simulink model "pend_MPC"  (R2018b)
settings: Solver=FixedStepAuto  StartTime=0.0  StopTime=30  FixedStep=h  RelTol=1e-3  EnableMultiTasking=on
PreLoadFcn:
  | hwinit
StartFcn:
  | hwinit
values from neighbouring files (symbols this model uses):
  adingain = [1, 1]    [hwinit.m]
  adinoffs = [-0.2676;-0.1653]    [hwinit.m]
  d_cart = X(1)    [main.m]
  d_pend = X_2(1)    [main.m]    (also in pend_par.m = x(1))
  daoutgain = [0.9]    [hwinit.m]
  daoutoffs = [0]    [hwinit.m]
  h = 0.01    [calib.m]    (also in main.m = 0.001; pend_par.m)
  Km = X(2)    [main.m]
  mc = X(3)    [main.m]
  mp = X_2(2)    [main.m]    (also in pend_par.m = x(2))
  option = 1    [main.m]
  T_final = 40    [main.m]
  x_init = [Pos_Pendulum.data(1),0,Angle_Pendulum.data(1),0]    [main.m]
undefined symbols (not defined in the file or in its folder): Advantech, angle_bound, angle_real, DiscIntNeverNeededParam, Discrete, dsys, K, kalman, l, PCI, pend, Time
libraries: simulink x2, sldrtlib x2, ctrlSharedLib x1, mpclib x1
settings Model: Creator=zhidayat  LastModifiedBy=dvanhanswijk
settings DataIOCC: LimitDataPoints=on  SaveFormat=Array
settings OptimizationCC: ExpressionDepthLimit=2147483647  LifeSpan=inf
settings DebuggingCC: AllowSymbolicDim=off  StateNameClashWarn=warning  StrictBusMsg=ErrorOnBusTreatedAsVector  SFUnexpectedBacktrackingDiag=warning  SFNoUnconditionalDefaultTransitionDiag=warning  SFExecutionAtInitializationDiag=none
settings HardwareCC: ProdBitPerPointer=32  ProdBitPerSizeT=32  ProdBitPerPtrDiffT=32  ProdLargestAtomicFloat=None  ProdIntDivRoundTo=Undefined  ProdEndianess=Unspecified  ProdWordSize=32  ProdHWDeviceType=32-bit Generic
settings ModelReferenceCC: PropagateSignalLabelsOutOfModel=off
settings SFSimCC: SimUseLocalCustomCode=off
settings RTWCC: RTWUseLocalCustomCode=off
settings CodeAppCC: StateflowObjectComments=on
settings GRTTargetCC: TargetLangStandard=C89/C90 (ANSI)  GeneratePreprocessorConditionals=Disable all  CombineOutputUpdateFcns=off  GRTInterface=on
settings ConfigComp: CovMetricSettings=dw  CovHtmlReporting=on  CovSaveCumulativeToWorkspaceVar=on  CovSaveSingleToWorkspaceVar=on  CovExternalEMLEnable=off

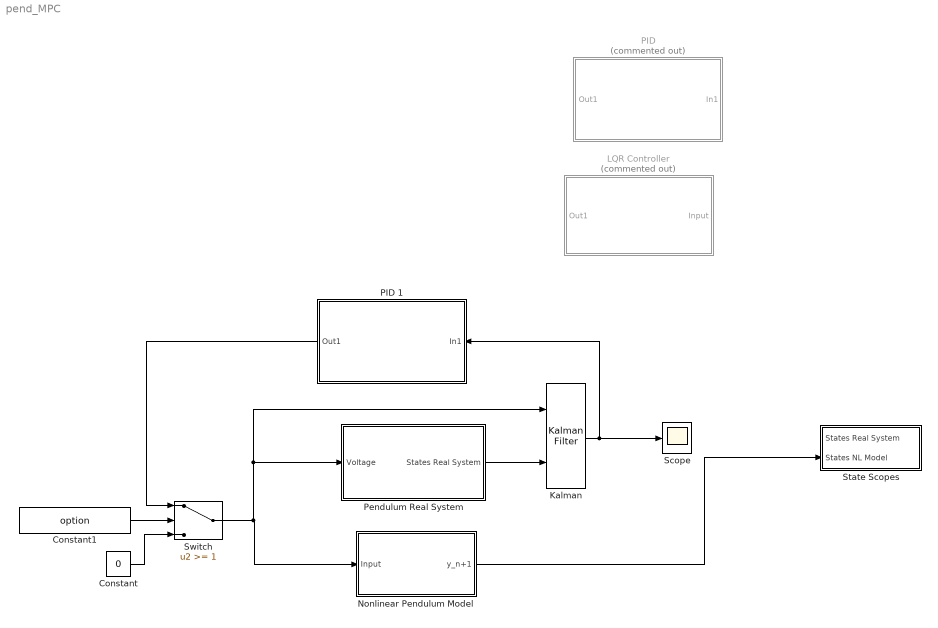
== system pend_MPC ==
  Constant : Constant  Value=0
  Constant1 : Constant  Value=option
  "Kalman " : ctrlSharedLib/Kalman Filter  TimeDomain=Discrete-Time  UseCurrentEstimator=on  ModelSource=Individual A, B, C, D matrices  ModelSourceVariable=ss(0.95,1,1,0,1)  A=dsys.A  B=dsys.B  C=dsys.C  D=dsys.D  NumberOfStates=4  NumberOfInputs=1  NumberOfOutputs=2  InitialEstimateSource=Dialog  X0=x_init  P0=10  UseK=off  UseGH=off  NumberOfProcessNoiseInputs=1  G=1  TimeInvariantG=on  H=0  TimeInvariantH=on  Q=kalman.Q  TimeInvariantQ=on  R=kalman.R  TimeInvariantR=on  N=0  TimeInvariantN=on  AddInputPort=on  AddEnablePort=off  OutputEstimatedY=off  OutputP=off  Ts=h
      settings: SourceProductBaseCode=CT
  LQR Controller : Subsystem  Commented=on
  Nonlinear Pendulum Model : Subsystem
  "PID " : Subsystem  Commented=on
  PID 1 : Subsystem
  "Pendulum Real System " : Subsystem
  Scope : Scope
  "State Scopes " : Subsystem
  Switch : Switch  Threshold=1
  wires:
  Nonlinear Pendulum Model/1(y_n+1) -> "State Scopes "/2(States NL Model)
  Constant/1 -> Switch/3
  Constant1/1 -> Switch/2
  "Pendulum Real System "/1(States Real System) -> "Kalman "/2
  PID 1/1(Out1) -> Switch/1
  Switch/1 -> Nonlinear Pendulum Model/1(Input), "Pendulum Real System "/1(Voltage), "Kalman "/1
  "Kalman "/1 -> Scope/1, PID 1/1(In1)

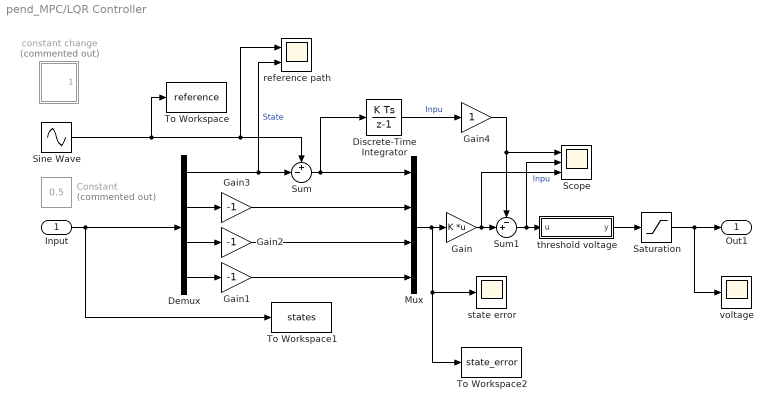
== system pend_MPC/LQR Controller ==
  Input : Inport
  Constant : Constant  Commented=on  Value=0.5
  Demux : Demux
  Discrete-Time Integrator : DiscreteIntegrator  gainval=1  SampleTime=h  ICPrevOutput=DiscIntNeverNeededParam  ICPrevScaledInput=DiscIntNeverNeededParam
  Gain : Gain  Gain=K  Multiplication=Matrix(K*u)
  Gain1 : Gain  Gain=-1
  Gain2 : Gain  Gain=-1
  Gain3 : Gain  Gain=-1
  Gain4 : Gain
  Mux : Mux
  Saturation : Saturate  UpperLimit=1  LowerLimit=-1
  Scope : Scope  NumInputPorts=3
  Sine Wave : Sin  Amplitude=0.1  Bias=0.5  SampleTime=h
  Sum : Sum  Inputs=+-|
  Sum1 : Sum  Inputs=-+|
  To Workspace : ToWorkspace  VariableName=reference  SaveFormat=Timeseries  SampleTime=-1
  To Workspace1 : ToWorkspace  VariableName=states  SaveFormat=Timeseries  SampleTime=-1
  To Workspace2 : ToWorkspace  VariableName=state_error  SaveFormat=Timeseries  SampleTime=-1
  "constant change " : Subsystem  Commented=on
  reference path : Scope  NumInputPorts=2
  state error : Scope
  threshold voltage : MATLAB Function  TreatAsAtomicUnit=on
  voltage : Scope
  Out1 : Outport
  wires:
  Input/1 -> To Workspace1/1, Demux/1
  Demux/2 -> Gain3/1
  Mux/1 -> Gain/1, To Workspace2/1, state error/1
  Demux/1 -> reference path/2, Sum/2  "State"
  Demux/3 -> Gain2/1
  Demux/4 -> Gain1/1
  threshold voltage/1(y) -> Saturation/1
  Sine Wave/1 -> To Workspace/1, reference path/1, Sum/1
  Gain/1 -> Scope/3, Sum1/2  "Inpu"
  Sum1/1 -> Scope/2, threshold voltage/1(u)
  Saturation/1 -> voltage/1, Out1/1
  Sum/1 -> Discrete-Time Integrator/1, Mux/1
  Gain3/1 -> Mux/2
  Gain2/1 -> Mux/3
  Gain1/1 -> Mux/4
  Discrete-Time Integrator/1 -> Gain4/1  "Inpu"
  Gain4/1 -> Scope/1, Sum1/1

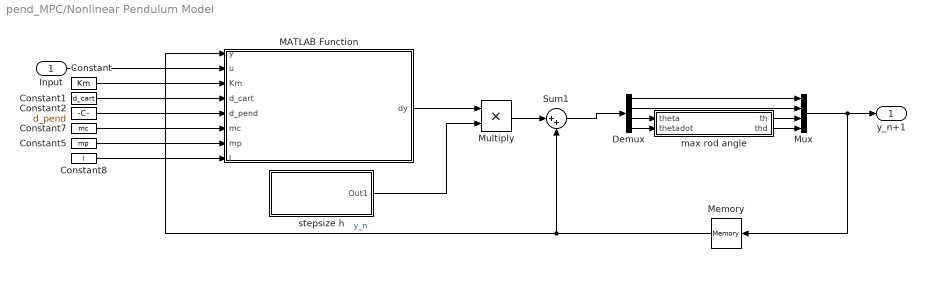
== system pend_MPC/Nonlinear Pendulum Model ==
  Input : Inport
  Constant : Constant  Value=Km
  Constant1 : Constant  Value=d_cart
  Constant2 : Constant  Value=d_pend
  Constant5 : Constant  Value=mp
  Constant7 : Constant  Value=mc
  Constant8 : Constant  Value=l  SampleTime=h
  Demux : Demux
  MATLAB Function : MATLAB Function  TreatAsAtomicUnit=on
  Memory : Memory  InitialCondition=x_init
  Multiply : Product
  Mux : Mux
  Sum1 : Sum  Inputs=|++
  max rod angle : MATLAB Function  TreatAsAtomicUnit=on
  stepsize h : Subsystem
  y_n+1 : Outport
  wires:
  Multiply/1 -> Sum1/1
  Memory/1 -> MATLAB Function/1(y), Sum1/2  "y_n"
  stepsize h/1(Out1) -> Multiply/2
  Constant/1 -> MATLAB Function/3(Km)
  Constant1/1 -> MATLAB Function/4(d_cart)
  Demux/2 -> Mux/2
  Demux/1 -> Mux/1
  Input/1 -> MATLAB Function/2(u)
  Constant2/1 -> MATLAB Function/5(d_pend)
  MATLAB Function/1(dy) -> Multiply/1
  Constant5/1 -> MATLAB Function/7(mp)
  Constant7/1 -> MATLAB Function/6(mc)
  Constant8/1 -> MATLAB Function/8(l)
  Demux/3 -> max rod angle/1(theta)
  Demux/4 -> max rod angle/2(thetadot)
  max rod angle/1(th) -> Mux/3
  max rod angle/2(thd) -> Mux/4
  Sum1/1 -> Demux/1
  Mux/1 -> Memory/1, y_n+1/1

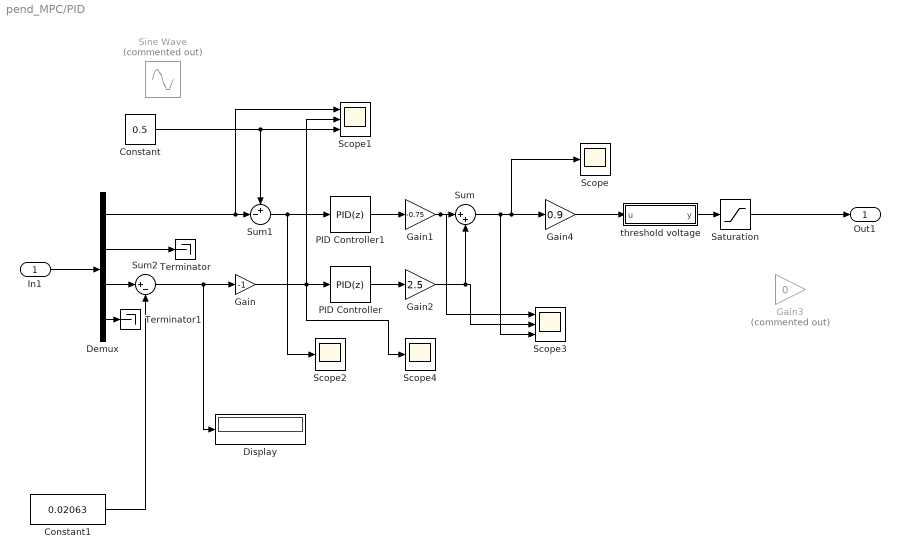
== system pend_MPC/PID  ==
  In1 : Inport
  Constant : Constant  Value=0.5
  Constant1 : Constant  Value=0.02063
  Demux : Demux
  Display : Display
  Gain : Gain  Gain=-1
  Gain1 : Gain  Gain=-0.75
  Gain2 : Gain  Gain=2.5
  Gain3 : Gain  Commented=on  Gain=0
  Gain4 : Gain  Gain=0.9
  PID Controller : simulink/Continuous/PID Controller  Controller=PID  Form=Parallel  TimeDomain=Discrete-time  SampleTime=h  IntegratorMethod=Forward Euler  FilterMethod=Forward Euler  ControllerParametersSource=internal  P=30  I=0  D=0.015  UseFilter=on  N=100  TunerSelectOption=Transfer Function Based (PID Tuner App)  InitialConditionSource=internal  InitialConditionForIntegrator=0  InitialConditionForFilter=0  DifferentiatorICPrevScaledInput=0  ExternalReset=none  TrackingMode=off  Kt=1  LimitOutput=off  UpperSaturationLimit=inf  LowerSaturationLimit=-inf  LinearizeAsGain=on  AntiWindupMode=none  Kb=1  POutMin=[]  POutMax=[]  IOutMin=[]  IOutMax=[]  DOutMin=[]  DOutMax=[]  NOutMin=[]  NOutMax=[]  SumOutMin=[]  SumOutMax=[]  SaturationOutMin=[]  SaturationOutMax=[]  PParamMin=[]  PParamMax=[]  IParamMin=[]  IParamMax=[]  DParamMin=[]  DParamMax=[]  NParamMin=[]  NParamMax=[]  KbParamMin=[]  KbParamMax=[]  KtParamMin=[]  KtParamMax=[]  KbOutMin=[]  KbOutMax=[]  KtOutMin=[]  KtOutMax=[]  IntegratorOutMin=[]  IntegratorOutMax=[]  FilterOutMin=[]  FilterOutMax=[]  SumI1OutMin=[]  SumI1OutMax=[]  SumI2OutMin=[]  SumI2OutMax=[]  SumI3OutMin=[]  SumI3OutMax=[]  SumI4OutMin=[]  SumI4OutMax=[]  SumDOutMin=[]  SumDOutMax=[]  DifferentiatorOutMin=[]  DifferentiatorOutMax=[]  FilterDiffOutCoefMin=[]  FilterDiffOutCoefMax=[]  ReciprocalOutMin=[]  ReciprocalOutMax=[]  SumDenOutMin=[]  SumDenOutMax=[]  SumNumOutMin=[]  SumNumOutMax=[]  DivideOutMin=[]  DivideOutMax=[]  IntegratorContinuousStateAttributes=''  IntegratorStateMustResolveToSignalObject=off  IntegratorRTWStateStorageClass=Auto  FilterContinuousStateAttributes=''  FilterStateMustResolveToSignalObject=off  FilterRTWStateStorageClass=Auto  ParallelPVariant=InternalParameters  IdealPVariant=Disabled  IVariant=InternalParameters  DVariant=InternalParameters  IntegratorVariant=Discrete  SatVariant=Disabled  AWVariant=Passthrough  PCopyVariant=Disabled  TRVariant=Disabled  FdbkBlocksVariant=Forward  IdealPFdbkVariant=Disabled  SatFdbkVariant=Disabled  DerivativeFilterVariant=ForwardEulerFilter  NVariant=InternalParameters  NCopyVariant=Disabled  FilterICVariant=InternalICsFilter  IntegratorICVariant=InternalICs  ExternalResetVariant=Disabled  TRSumVariant=Passthrough  SumFdbkVariant=Disabled  SumVariant=Sum_PID
  PID Controller1 : simulink/Continuous/PID Controller  Controller=PID  Form=Parallel  TimeDomain=Discrete-time  SampleTime=h  IntegratorMethod=Forward Euler  FilterMethod=Forward Euler  ControllerParametersSource=internal  P=13  I=0.75  D=0.75  UseFilter=on  N=100  TunerSelectOption=Transfer Function Based (PID Tuner App)  InitialConditionSource=internal  InitialConditionForIntegrator=0  InitialConditionForFilter=0  DifferentiatorICPrevScaledInput=0  ExternalReset=none  TrackingMode=off  Kt=1  LimitOutput=off  UpperSaturationLimit=inf  LowerSaturationLimit=-inf  LinearizeAsGain=on  AntiWindupMode=none  Kb=1  POutMin=[]  POutMax=[]  IOutMin=[]  IOutMax=[]  DOutMin=[]  DOutMax=[]  NOutMin=[]  NOutMax=[]  SumOutMin=[]  SumOutMax=[]  SaturationOutMin=[]  SaturationOutMax=[]  PParamMin=[]  PParamMax=[]  IParamMin=[]  IParamMax=[]  DParamMin=[]  DParamMax=[]  NParamMin=[]  NParamMax=[]  KbParamMin=[]  KbParamMax=[]  KtParamMin=[]  KtParamMax=[]  KbOutMin=[]  KbOutMax=[]  KtOutMin=[]  KtOutMax=[]  IntegratorOutMin=[]  IntegratorOutMax=[]  FilterOutMin=[]  FilterOutMax=[]  SumI1OutMin=[]  SumI1OutMax=[]  SumI2OutMin=[]  SumI2OutMax=[]  SumI3OutMin=[]  SumI3OutMax=[]  SumI4OutMin=[]  SumI4OutMax=[]  SumDOutMin=[]  SumDOutMax=[]  DifferentiatorOutMin=[]  DifferentiatorOutMax=[]  FilterDiffOutCoefMin=[]  FilterDiffOutCoefMax=[]  ReciprocalOutMin=[]  ReciprocalOutMax=[]  SumDenOutMin=[]  SumDenOutMax=[]  SumNumOutMin=[]  SumNumOutMax=[]  DivideOutMin=[]  DivideOutMax=[]  IntegratorContinuousStateAttributes=''  IntegratorStateMustResolveToSignalObject=off  IntegratorRTWStateStorageClass=Auto  FilterContinuousStateAttributes=''  FilterStateMustResolveToSignalObject=off  FilterRTWStateStorageClass=Auto  ParallelPVariant=InternalParameters  IdealPVariant=Disabled  IVariant=InternalParameters  DVariant=InternalParameters  IntegratorVariant=Discrete  SatVariant=Disabled  AWVariant=Passthrough  PCopyVariant=Disabled  TRVariant=Disabled  FdbkBlocksVariant=Forward  IdealPFdbkVariant=Disabled  SatFdbkVariant=Disabled  DerivativeFilterVariant=ForwardEulerFilter  NVariant=InternalParameters  NCopyVariant=Disabled  FilterICVariant=InternalICsFilter  IntegratorICVariant=InternalICs  ExternalResetVariant=Disabled  TRSumVariant=Passthrough  SumFdbkVariant=Disabled  SumVariant=Sum_PID
  Saturation : Saturate  UpperLimit=1  LowerLimit=-1
  Scope : Scope
  Scope1 : Scope  NumInputPorts=3
  Scope2 : Scope
  Scope3 : Scope  NumInputPorts=3
  Scope4 : Scope
  Sine Wave : Sin  Commented=on  Amplitude=0.15  Bias=0.5  Frequency=0.5  SampleTime=h
  Sum : Sum  Inputs=|++
  Sum1 : Sum  Inputs=+-|
  Sum2 : Sum  Inputs=|+-
  Terminator : Terminator
  Terminator1 : Terminator
  threshold voltage : MATLAB Function  TreatAsAtomicUnit=on
  Out1 : Outport
  wires:
  Demux/2 -> Terminator/1
  Demux/4 -> Terminator1/1
  PID Controller1/1 -> Gain1/1
  Sum/1 -> Scope3/3, Scope/1, Gain4/1
  In1/1 -> Demux/1
  PID Controller/1 -> Gain2/1
  Demux/1 -> Scope1/1, Sum1/2
  Constant/1 -> Scope1/3, Sum1/1
  Sum1/1 -> Scope2/1, PID Controller1/1
  Gain1/1 -> Scope3/1, Sum/1
  Gain2/1 -> Scope3/2, Sum/2
  threshold voltage/1(y) -> Saturation/1
  Sum2/1 -> Gain/1, Display/1
  Saturation/1 -> Out1/1
  Demux/3 -> Sum2/1
  Constant1/1 -> Sum2/2
  Gain/1 -> Scope1/2, PID Controller/1, Scope4/1
  Gain4/1 -> threshold voltage/1(u)

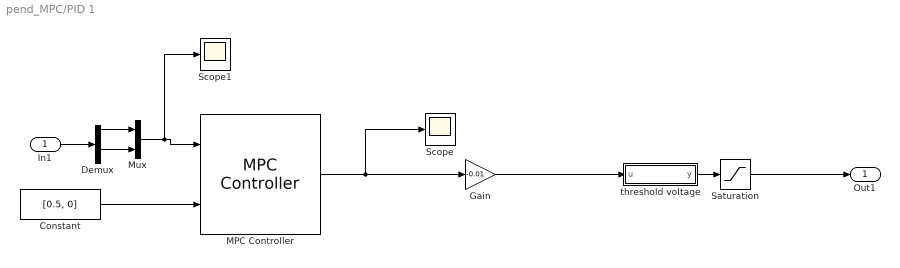
== system pend_MPC/PID 1 ==
  In1 : Inport
  Constant : Constant  Value=[0.5, 0]
  Demux : Demux
  Gain : Gain  Gain=-0.01
  MPC Controller : mpclib/MPC Controller  SCDEnableBlockLinearizationSpecification=on  mpcobj=MPCOBJ  is_multiple=0  enable_value=0  return_u0=off  updateMPCinCallerWorkspace=on  md_inport=off  mv_inport=off  return_cost=off  return_mvseq=off  return_qpstatus=off  return_xseq=off  return_state=off  return_ovseq=off  state_inport=off  umin_inport=off  umax_inport=off  ymin_inport=off  ymax_inport=off  cc_inport=off  ywt_inport=off  uwt_inport=off  duwt_inport=off  rhoeps_inport=off  uref_inport=off  n_ts=0.001  n_p=10  n_mv=1  n_md=0  n_ud=0  n_mo=2  n_uo=0  BlockDataType=double  SampleTimeInherited=off  switch_inport=off
  Mux : Mux  Inputs=2
  Saturation : Saturate  UpperLimit=1  LowerLimit=-1
  Scope : Scope
  Scope1 : Scope
  threshold voltage : MATLAB Function  TreatAsAtomicUnit=on
  Out1 : Outport
  wires:
  threshold voltage/1(y) -> Saturation/1
  Saturation/1 -> Out1/1
  Constant/1 -> MPC Controller/2
  Gain/1 -> threshold voltage/1(u)
  In1/1 -> Demux/1
  Demux/1 -> Mux/1
  Demux/3 -> Mux/2
  Mux/1 -> Scope1/1, MPC Controller/1
  MPC Controller/1 -> Scope/1, Gain/1

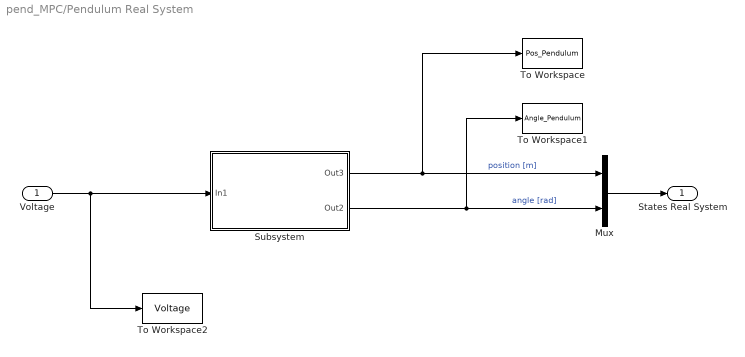
== system pend_MPC/Pendulum Real System  ==
  Voltage : Inport
  Mux : Mux  Inputs=2
  Subsystem : Subsystem  InitFcn=hwinit  StartFcn=hwinit  mask{h=h}
      mask prompts: h "Sample time"
      mask init:
      | hwinit
      mask Display: disp('Pendulum');
  To Workspace : ToWorkspace  VariableName=Pos_Pendulum  SaveFormat=Timeseries  SampleTime=-1
  To Workspace1 : ToWorkspace  VariableName=Angle_Pendulum  SaveFormat=Timeseries  SampleTime=-1
  To Workspace2 : ToWorkspace  VariableName=Voltage  SaveFormat=Timeseries  SampleTime=-1
  States Real System : Outport
  wires:
  Voltage/1 -> To Workspace2/1, Subsystem/1(In1)
  Subsystem/1(Out3) -> To Workspace/1, Mux/1  "position [m]"
  Subsystem/2(Out2) -> Mux/2, To Workspace1/1  "angle [rad]"
  Mux/1 -> States Real System/1

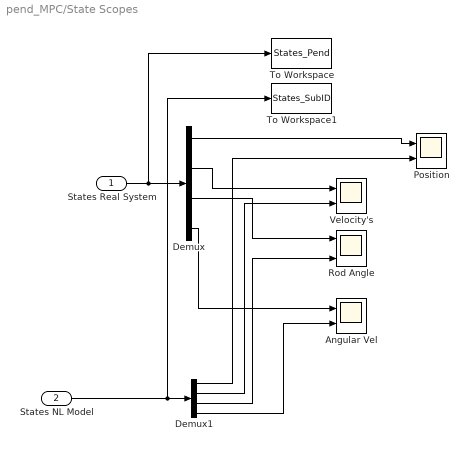
== system pend_MPC/State Scopes  ==
  States Real System : Inport
  States NL Model : Inport  Port=2
  "Angular Vel " : Scope  NumInputPorts=2
  Demux : Demux
  Demux1 : Demux
  Position : Scope  NumInputPorts=2
  Rod Angle : Scope  NumInputPorts=2
  To Workspace : ToWorkspace  VariableName=States_Pend  SaveFormat=Timeseries  SampleTime=-1
  To Workspace1 : ToWorkspace  VariableName=States_SubID  SaveFormat=Timeseries  SampleTime=h
  Velocity's : Scope  NumInputPorts=2
  wires:
  States Real System/1 -> To Workspace/1, Demux/1
  Demux/1 -> Position/1
  States NL Model/1 -> To Workspace1/1, Demux1/1
  Demux1/2 -> Velocity's/2
  Demux/2 -> Velocity's/1
  Demux/3 -> Rod Angle/1
  Demux1/3 -> Rod Angle/2
  Demux/4 -> "Angular Vel "/1
  Demux1/4 -> "Angular Vel "/2
  Demux1/1 -> Position/2

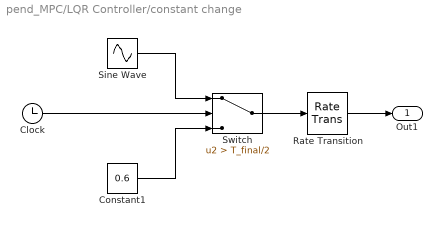
== system pend_MPC/LQR Controller/constant change  ==
  Clock : Clock
  Constant1 : Constant  Value=0.6
  Rate Transition : RateTransition  OutPortSampleTime=h
  Sine Wave : Sin  Amplitude=0.2  Bias=0.5  SampleTime=h
  Switch : Switch  Criteria=u2 > Threshold  Threshold=T_final/2
  Out1 : Outport
  wires:
  Sine Wave/1 -> Switch/1
  Constant1/1 -> Switch/3
  Clock/1 -> Switch/2
  Switch/1 -> Rate Transition/1
  Rate Transition/1 -> Out1/1

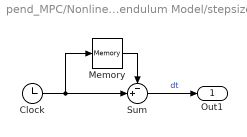
== system pend_MPC/Nonlinear Pendulum Model/stepsize h ==
  Clock : Clock
  Memory : Memory
  Sum : Sum  Inputs=-+|
  Out1 : Outport
  wires:
  Memory/1 -> Sum/1
  Sum/1 -> Out1/1  "dt"
  Clock/1 -> Memory/1, Sum/2

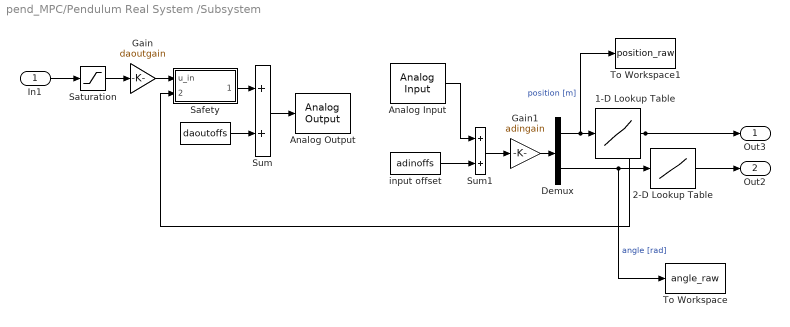
== system pend_MPC/Pendulum Real System /Subsystem ==
  In1 : Inport
  " " : Constant  Value=daoutoffs
  1-D Lookup Table : Lookup_n-D  NumberOfTableDimensions=1  BreakpointsForDimension1=pend  Table=real  InternalRulePriority=Speed  RndMeth=Simplest  InputSameDT=on
  2-D Lookup Table : Lookup_n-D  NumberOfTableDimensions=1  BreakpointsForDimension1=angle_real  BreakpointsForDimension2=[1:3]  Table=angle_bound  InternalRulePriority=Speed  RndMeth=Simplest  InputSameDT=on
  Analog Input : sldrtlib/Analog Input  SampleTime=h  MaxMissedTicks=ticklost  ShowMissedTicks=off  YieldWhenWaiting=on  DrvName=Advantech/PCI-1711  DrvAddress=4294967295  DrvOptions=zeros(1,0)  Channels=adinchannels  RangeMode=2  VoltRange=1  DataType=1
      settings: AttributesFormatString=Advantech\nPCI-1711 [auto]  SourceProductName=Simulink Desktop Real-Time
  Analog Output : sldrtlib/Analog Output  SampleTime=h  MaxMissedTicks=ticklost  ShowMissedTicks=off  YieldWhenWaiting=off  DrvName=Advantech/PCI-1711  DrvAddress=4294967295  DrvOptions=zeros(1,0)  Channels=daoutchannels  RangeMode=2  VoltRange=2  InitialValue=0  FinalValue=0
      settings: AttributesFormatString=Advantech\nPCI-1711 [auto]  SourceProductName=Simulink Desktop Real-Time
  Demux : Demux  Outputs=2
  Gain : Gain  Gain=daoutgain  SaturateOnIntegerOverflow=on  OutDataTypeStr=Inherit: Same as input  ParamDataTypeStr=Inherit: Same as input
  Gain1 : Gain  Gain=adingain  SaturateOnIntegerOverflow=on  OutDataTypeStr=Inherit: Same as input  ParamDataTypeStr=Inherit: Same as input
  Safety : Subsystem
      mask help: The output of the block is restricted to prevent damage to the system. If the cart reaches some safety margins (left: -0.26 and right: 0.26), the output of the block is nullifed. Then the control has to be restarted.
      mask Display: disp('Safety \n margins')
  Saturation : Saturate  UpperLimit=1  LowerLimit=-1
  Sum : Sum  SaturateOnIntegerOverflow=on  OutDataTypeStr=Inherit: Same as first input
  Sum1 : Sum  SaturateOnIntegerOverflow=on  InputSameDT=on  OutDataTypeStr=Inherit: Same as first input
  To Workspace : ToWorkspace  VariableName=angle_raw  SaveFormat=Timeseries  SampleTime=-1
  To Workspace1 : ToWorkspace  VariableName=position_raw  SaveFormat=Timeseries  SampleTime=-1
  input offset : Constant  Value=adinoffs
  Out3 : Outport
  Out2 : Outport  Port=2
  wires:
  Sum1/1 -> Gain1/1
  input offset/1 -> Sum1/2
  Analog Input/1 -> Sum1/1
  Gain1/1 -> Demux/1
  Saturation/1 -> Gain/1
  Sum/1 -> Analog Output/1
  " "/1 -> Sum/2
  In1/1 -> Saturation/1
  Demux/2 -> 2-D Lookup Table/1, To Workspace/1  "angle [rad]"
  Safety/1(u_out) -> Sum/1
  Gain/1 -> Safety/1(u_in)
  Demux/1 -> To Workspace1/1, 1-D Lookup Table/1  "position [m]"
  1-D Lookup Table/1 -> Safety/2(Position), Out3/1
  2-D Lookup Table/1 -> Out2/1

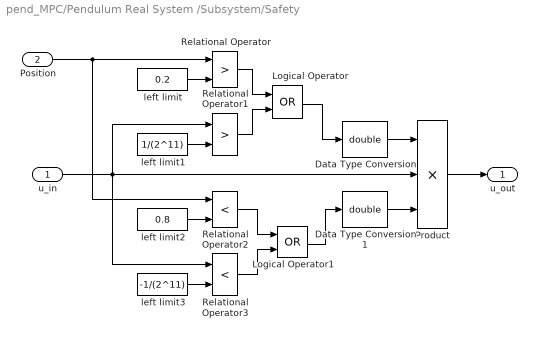
== system pend_MPC/Pendulum Real System /Subsystem/Safety ==
  u_in : Inport
  Position : Inport  Port=2
  Data Type Conversion : DataTypeConversion  OutDataTypeStr=double
  Data Type Conversion1 : DataTypeConversion  OutDataTypeStr=double
  Logical Operator : Logic  Operator=OR  OutDataTypeStr=boolean
  Logical Operator1 : Logic  Operator=OR  OutDataTypeStr=boolean
  Product : Product  Inputs=3  SaturateOnIntegerOverflow=on  InputSameDT=on  OutDataTypeStr=Inherit: Same as first input
  Relational Operator : RelationalOperator  Operator=>  OutDataTypeStr=boolean  RndMeth=Nearest  InputSameDT=on
  Relational Operator1 : RelationalOperator  Operator=>  OutDataTypeStr=boolean  RndMeth=Nearest  InputSameDT=on
  Relational Operator2 : RelationalOperator  Operator=<  OutDataTypeStr=boolean  RndMeth=Nearest  InputSameDT=on
  Relational Operator3 : RelationalOperator  Operator=<  OutDataTypeStr=boolean  RndMeth=Nearest  InputSameDT=on
  left limit : Constant  Value=0.2
  left limit1 : Constant  Value=1/(2^11)
  left limit2 : Constant  Value=0.8
  left limit3 : Constant  Value=-1/(2^11)
  u_out : Outport
  wires:
  left limit1/1 -> Relational Operator1/2
  u_in/1 -> Relational Operator1/1, Relational Operator3/1, Product/2
  Logical Operator1/1 -> Data Type Conversion1/1
  Logical Operator/1 -> Data Type Conversion/1
  left limit/1 -> Relational Operator/2
  Relational Operator/1 -> Logical Operator/1
  Relational Operator1/1 -> Logical Operator/2
  Position/1 -> Relational Operator/1, Relational Operator2/1
  left limit2/1 -> Relational Operator2/2
  Relational Operator2/1 -> Logical Operator1/1
  left limit3/1 -> Relational Operator3/2
  Relational Operator3/1 -> Logical Operator1/2
  Product/1 -> u_out/1
  Data Type Conversion/1 -> Product/1
  Data Type Conversion1/1 -> Product/3

== matlab function pend_MPC/LQR Controller/threshold voltage ==
  data: u input; y output
function y = fcn(u)
ub_mtr_threshold = 0.26;
       y = u + sign(u)*0.9*ub_mtr_threshold;
%        if abs(u) <= ub_mtr_threshold && abs(u) >= lb_mtr_threshold
%            y = sign(u)*(ub_mtr_threshold + 0.02);
%        elseif abs(u) <= lb_mtr_threshold
%            y = 0;
%        else 
%            y = u;
%        end
end

== matlab function pend_MPC/Nonlinear Pendulum Model/MATLAB Function ==
  data: y input; u input; dy output; Km input; d_cart input; d_pend input; mc input; mp input; l input
function dy = nl_pend_dynamics(y,u,Km,d_cart,d_pend,mc,mp,l)
g = 9.81;
dy = zeros(4,1);

dy(1,1) = y(2);
dy(2,1) = 1/((mc+mp)*(1-0.75*mp))*(Km*u - d_cart*y(2) + 3/(2*l)*((l/2)*mp*g*y(3) - d_pend*y(4)) + mp*l*y(4)^2*y(3)/2);
dy(3,1) = y(4);
dy(4,1) = 3/(mp*l^2)*(l*mp*dy(2,1)/2 + l*mp*g*y(3)/2 - d_pend*y(4));

== matlab function pend_MPC/PID /threshold voltage ==
  data: u input; y output
function y = fcn(u)
ub_mtr_threshold = 0.26;
       y = u + sign(u)*0.9*ub_mtr_threshold;
%        if abs(u) <= ub_mtr_threshold && abs(u) >= lb_mtr_threshold
%            y = sign(u)*(ub_mtr_threshold + 0.02);
%        elseif abs(u) <= lb_mtr_threshold
%            y = 0;
%        else 
%            y = u;
%        end
end

== matlab function pend_MPC/Nonlinear Pendulum Model/max rod angle ==
  data: theta input; th output; thetadot input; thd output
function [th,thd] = fcn(theta, thetadot)
threshold = 0.26;

if abs(theta) > threshold
    th = threshold*sign(theta);
    thd = 0;
else
    th = theta;
    thd = thetadot;
end

== matlab function pend_MPC/PID 1/threshold voltage ==
  data: u input; y output
function y = fcn(u)
ub_mtr_threshold = 0.26;
       y = u + sign(u)*0.9*ub_mtr_threshold;
%        if abs(u) <= ub_mtr_threshold && abs(u) >= lb_mtr_threshold
%            y = sign(u)*(ub_mtr_threshold + 0.02);
%        elseif abs(u) <= lb_mtr_threshold
%            y = 0;
%        else 
%            y = u;
%        end
end
